simulink model "uavPackageDelivery_3UAV_photo3D_test"  (R2026a)
settings: Solver=VariableStepAuto  StopTime=20  FixedStep=.005  EnableMultiTasking=on
undefined symbols (not defined in the file or in its folder): baseMission, Newton, oaMission, Raphson, uavIC_latLon, UAVSampleTime
libraries: robotcorelib x3, uavalgslib x3, robotalgslib x3, simulink x2
(part 2 of 2)

== system uavPackageDelivery_3UAV_photo3D_test/OnBoard_UAV1/DataProcessing/ProcessSensorData/Compute Ranges/For Each Subsystem ==
  In1 : Inport  Partition=on  PartitionDimension=1  PartitionWidth=1  PartitionOffset=0
  For Each : ForEach  DisableCoverage=on
  Product : Product
  Product1 : Product
  Selector : Selector  InputPortWidth=3  IndexOptions=Index vector (dialog)  Indices=[1]  OutputSizes=1
  Selector1 : Selector  InputPortWidth=3  IndexOptions=Index vector (dialog)  Indices=[2]  OutputSizes=1
  Sqrt : Sqrt  OutputSignalType=real  OutDataTypeStr=single  IntermediateResultsDataTypeStr=single  AlgorithmType=Newton-Raphson
  Sum : Sum  Inputs=|++
  Out1 : Outport  ConcatenationDimension=1
  wires:
  In1/1 -> Selector1/1, Selector/1
  Selector/1 -> Product/2, Product/1
  Selector1/1 -> Product1/2, Product1/1
  Product/1 -> Sum/1
  Product1/1 -> Sum/2
  Sum/1 -> Sqrt/1
  Sqrt/1 -> Out1/1

== system uavPackageDelivery_3UAV_photo3D_test/OnBoard_UAV2/DataProcessing/Process3DSensorData/Compute Ranges/For Each Subsystem1 ==
  In1 : Inport  Partition=on  PartitionDimension=1  PartitionWidth=1  PartitionOffset=0
  For Each Horizontal Slice : ForEach  DisableCoverage=on
  Process each Horizontal Slice : Subsystem  TreatAsAtomicUnit=on
  Reshape : Reshape
  Out1 : Outport  ConcatenationDimension=1
  wires:
  In1/1 -> Process each Horizontal Slice/1(pointCloud)
  Process each Horizontal Slice/1(Out1) -> Reshape/1
  Reshape/1 -> Out1/1

== system uavPackageDelivery_3UAV_photo3D_test/OnBoard_UAV2/DataProcessing/ProcessSensorData/Compute Ranges/For Each Subsystem ==
  In1 : Inport  Partition=on  PartitionDimension=1  PartitionWidth=1  PartitionOffset=0
  For Each : ForEach  DisableCoverage=on
  Product : Product
  Product1 : Product
  Selector : Selector  InputPortWidth=3  IndexOptions=Index vector (dialog)  Indices=[1]  OutputSizes=1
  Selector1 : Selector  InputPortWidth=3  IndexOptions=Index vector (dialog)  Indices=[2]  OutputSizes=1
  Sqrt : Sqrt  OutputSignalType=real  OutDataTypeStr=single  IntermediateResultsDataTypeStr=single  AlgorithmType=Newton-Raphson
  Sum : Sum  Inputs=|++
  Out1 : Outport  ConcatenationDimension=1
  wires:
  In1/1 -> Selector1/1, Selector/1
  Selector/1 -> Product/2, Product/1
  Selector1/1 -> Product1/2, Product1/1
  Product/1 -> Sum/1
  Product1/1 -> Sum/2
  Sum/1 -> Sqrt/1
  Sqrt/1 -> Out1/1

== system uavPackageDelivery_3UAV_photo3D_test/OnBoard_UAV3/DataProcessing/Process3DSensorData/Compute Ranges/For Each Subsystem1 ==
  In1 : Inport  Partition=on  PartitionDimension=1  PartitionWidth=1  PartitionOffset=0
  For Each Horizontal Slice : ForEach  DisableCoverage=on
  Process each Horizontal Slice : Subsystem  TreatAsAtomicUnit=on
  Reshape : Reshape
  Out1 : Outport  ConcatenationDimension=1
  wires:
  In1/1 -> Process each Horizontal Slice/1(pointCloud)
  Process each Horizontal Slice/1(Out1) -> Reshape/1
  Reshape/1 -> Out1/1

== system uavPackageDelivery_3UAV_photo3D_test/OnBoard_UAV3/DataProcessing/ProcessSensorData/Compute Ranges/For Each Subsystem ==
  In1 : Inport  Partition=on  PartitionDimension=1  PartitionWidth=1  PartitionOffset=0
  For Each : ForEach  DisableCoverage=on
  Product : Product
  Product1 : Product
  Selector : Selector  InputPortWidth=3  IndexOptions=Index vector (dialog)  Indices=[1]  OutputSizes=1
  Selector1 : Selector  InputPortWidth=3  IndexOptions=Index vector (dialog)  Indices=[2]  OutputSizes=1
  Sqrt : Sqrt  OutputSignalType=real  OutDataTypeStr=single  IntermediateResultsDataTypeStr=single  AlgorithmType=Newton-Raphson
  Sum : Sum  Inputs=|++
  Out1 : Outport  ConcatenationDimension=1
  wires:
  In1/1 -> Selector1/1, Selector/1
  Selector/1 -> Product/2, Product/1
  Selector1/1 -> Product1/2, Product1/1
  Product/1 -> Sum/1
  Product1/1 -> Sum/2
  Sum/1 -> Sqrt/1
  Sqrt/1 -> Out1/1

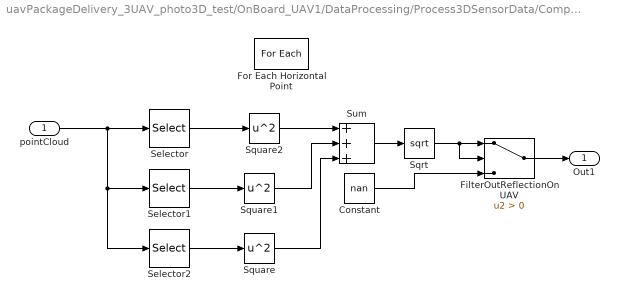
== system uavPackageDelivery_3UAV_photo3D_test/OnBoard_UAV1/DataProcessing/Process3DSensorData/Compute Ranges/For Each Subsystem1/Process each Horizontal Slice ==
  pointCloud : Inport  Partition=on  PartitionDimension=2  PartitionWidth=1  PartitionOffset=0
  Constant : Constant  Value=nan
  FilterOutReflectionOnUAV : Switch  Criteria=u2 > Threshold  SaturateOnIntegerOverflow=off  InputSameDT=off
  For Each Horizontal Point : ForEach  DisableCoverage=on
  Selector : Selector  NumberOfDimensions=3  InputPortWidth=3  IndexOptions=Index vector (dialog),Index vector (dialog),Index vector (dialog)  Indices=1,1,1  OutputSizes=1,1,1
  Selector1 : Selector  NumberOfDimensions=3  InputPortWidth=3  IndexOptions=Index vector (dialog),Index vector (dialog),Index vector (dialog)  Indices=1,1,2  OutputSizes=1,1,1
  Selector2 : Selector  NumberOfDimensions=3  InputPortWidth=3  IndexOptions=Index vector (dialog),Index vector (dialog),Index vector (dialog)  Indices=1,1,3  OutputSizes=1,1,1
  Sqrt : Sqrt  OutputSignalType=real  OutDataTypeStr=single  IntermediateResultsDataTypeStr=single  AlgorithmType=Newton-Raphson
  Square : Math  Operator=square
  Square1 : Math  Operator=square
  Square2 : Math  Operator=square
  Sum : Sum  Inputs=+++
  Out1 : Outport  ConcatenationDimension=1
  wires:
  pointCloud/1 -> Selector2/1, Selector1/1, Selector/1
  Selector/1 -> Square2/1
  Selector1/1 -> Square1/1
  Square2/1 -> Sum/1
  Square1/1 -> Sum/2
  Sum/1 -> Sqrt/1
  Sqrt/1 -> FilterOutReflectionOnUAV/1, FilterOutReflectionOnUAV/2
  Selector2/1 -> Square/1
  Square/1 -> Sum/3
  FilterOutReflectionOnUAV/1 -> Out1/1
  Constant/1 -> FilterOutReflectionOnUAV/3

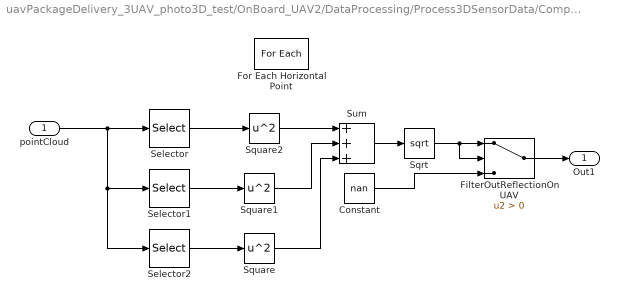
== system uavPackageDelivery_3UAV_photo3D_test/OnBoard_UAV2/DataProcessing/Process3DSensorData/Compute Ranges/For Each Subsystem1/Process each Horizontal Slice ==
  pointCloud : Inport  Partition=on  PartitionDimension=2  PartitionWidth=1  PartitionOffset=0
  Constant : Constant  Value=nan
  FilterOutReflectionOnUAV : Switch  Criteria=u2 > Threshold  SaturateOnIntegerOverflow=off  InputSameDT=off
  For Each Horizontal Point : ForEach  DisableCoverage=on
  Selector : Selector  NumberOfDimensions=3  InputPortWidth=3  IndexOptions=Index vector (dialog),Index vector (dialog),Index vector (dialog)  Indices=1,1,1  OutputSizes=1,1,1
  Selector1 : Selector  NumberOfDimensions=3  InputPortWidth=3  IndexOptions=Index vector (dialog),Index vector (dialog),Index vector (dialog)  Indices=1,1,2  OutputSizes=1,1,1
  Selector2 : Selector  NumberOfDimensions=3  InputPortWidth=3  IndexOptions=Index vector (dialog),Index vector (dialog),Index vector (dialog)  Indices=1,1,3  OutputSizes=1,1,1
  Sqrt : Sqrt  OutputSignalType=real  OutDataTypeStr=single  IntermediateResultsDataTypeStr=single  AlgorithmType=Newton-Raphson
  Square : Math  Operator=square
  Square1 : Math  Operator=square
  Square2 : Math  Operator=square
  Sum : Sum  Inputs=+++
  Out1 : Outport  ConcatenationDimension=1
  wires:
  pointCloud/1 -> Selector2/1, Selector1/1, Selector/1
  Selector/1 -> Square2/1
  Selector1/1 -> Square1/1
  Square2/1 -> Sum/1
  Square1/1 -> Sum/2
  Sum/1 -> Sqrt/1
  Sqrt/1 -> FilterOutReflectionOnUAV/1, FilterOutReflectionOnUAV/2
  Selector2/1 -> Square/1
  Square/1 -> Sum/3
  FilterOutReflectionOnUAV/1 -> Out1/1
  Constant/1 -> FilterOutReflectionOnUAV/3

== system uavPackageDelivery_3UAV_photo3D_test/OnBoard_UAV3/DataProcessing/Process3DSensorData/Compute Ranges/For Each Subsystem1/Process each Horizontal Slice ==
  pointCloud : Inport  Partition=on  PartitionDimension=2  PartitionWidth=1  PartitionOffset=0
  Constant : Constant  Value=nan
  FilterOutReflectionOnUAV : Switch  Criteria=u2 > Threshold  SaturateOnIntegerOverflow=off  InputSameDT=off
  For Each Horizontal Point : ForEach  DisableCoverage=on
  Selector : Selector  NumberOfDimensions=3  InputPortWidth=3  IndexOptions=Index vector (dialog),Index vector (dialog),Index vector (dialog)  Indices=1,1,1  OutputSizes=1,1,1
  Selector1 : Selector  NumberOfDimensions=3  InputPortWidth=3  IndexOptions=Index vector (dialog),Index vector (dialog),Index vector (dialog)  Indices=1,1,2  OutputSizes=1,1,1
  Selector2 : Selector  NumberOfDimensions=3  InputPortWidth=3  IndexOptions=Index vector (dialog),Index vector (dialog),Index vector (dialog)  Indices=1,1,3  OutputSizes=1,1,1
  Sqrt : Sqrt  OutputSignalType=real  OutDataTypeStr=single  IntermediateResultsDataTypeStr=single  AlgorithmType=Newton-Raphson
  Square : Math  Operator=square
  Square1 : Math  Operator=square
  Square2 : Math  Operator=square
  Sum : Sum  Inputs=+++
  Out1 : Outport  ConcatenationDimension=1
  wires:
  pointCloud/1 -> Selector2/1, Selector1/1, Selector/1
  Selector/1 -> Square2/1
  Selector1/1 -> Square1/1
  Square2/1 -> Sum/1
  Square1/1 -> Sum/2
  Sum/1 -> Sqrt/1
  Sqrt/1 -> FilterOutReflectionOnUAV/1, FilterOutReflectionOnUAV/2
  Selector2/1 -> Square/1
  Square/1 -> Sum/3
  FilterOutReflectionOnUAV/1 -> Out1/1
  Constant/1 -> FilterOutReflectionOnUAV/3

== matlab function uavPackageDelivery_3UAV_photo3D_test/GroundControl_UAV2/Get Flight Mission/QGC/Create Mission for Path Manager ==
  data: baseMission input Bus: uavPathManagerBus size=42; isNew input size=1; LTPMission input size=[42 3]; mission output Bus: uavPathManagerBus size=42; qgcMission input Bus: uavPathManagerBus size=42
function mission = generateWaypointStream(baseMission, isNew, LTPMission, qgcMission)

persistent UAVMission

if isempty(UAVMission)
    UAVMission = baseMission;
end

%% If we got a new mission
if (isNew == true)
   for ii=1:42
       if LTPMission(ii,2) < 7275326
           UAVMission(ii).position = LTPMission(ii,:)';
           y = isnan(qgcMission(ii).params);
           UAVMission(ii).params = qgcMission(ii).params;
           if sum(y)>0
               UAVMission(ii).params(y) = single(0);
           end
           UAVMission(ii).mode = mavlinkToPlannerType(qgcMission(ii).mode);
       end
   end
end

mission = UAVMission;

end

function plannerType =  mavlinkToPlannerType (mavlinkType)
% see enum name="MAV_CMD" in common.xml for values.
    switch mavlinkType
        case 16 %MAV_CMD_NAV_WAYPOINT
            plannerType = uint8(2);
        case 18 %MAV_CMD_NAV_LOITER_TURNS
            plannerType = uint8(3);
        case 21 %MAV_CMD_NAV_LAND
            plannerType = uint8(4);
        case 22 %MAV_CMD_NAV_TAKEOFF
            plannerType = uint8(1);
        otherwise %this will likely error out to signal something unexpected
            plannerType = uint8(0);
    end
end

== matlab function uavPackageDelivery_3UAV_photo3D_test/OnBoard_UAV2/DataProcessing/Process3DSensorData/ObstacleAvoidance/ReshapePointCloud ==
  data: u input; y output
function y = fcn(u)
y = [reshape(u(:,:,1),[],1), reshape(u(:,:,2),[],1), reshape(u(:,:,3),[],1)];

== matlab function uavPackageDelivery_3UAV_photo3D_test/OnBoard_UAV2/DataProcessing/Process3DSensorData/Visualize Front-Facing Camera ==
  data: imageFrame input
function plotImageFrame(imageFrame)

coder.extrinsic('ishandle','image');

persistent fig;

if isempty(fig)
    fig = figure();
    ax = newplot(fig);
    title(ax, 'Front-facing camera');
end

if ~isempty(fig) && ishandle(fig)
    ax = newplot(fig);
    image(ax, imageFrame);
    axis(ax, 'off');
end

== matlab function uavPackageDelivery_3UAV_photo3D_test/OnBoard_UAV2/DataProcessing/Process3DSensorData/Visualize Point cloud ==
  data: xyzPoints input
function VisualizePointCloud(xyzPoints)
%VisualizePointCloud Display point cloud

coder.extrinsic('isOpen', 'pcplayer')

persistent player;

if isempty(player)
    % Configure axes limits
    xlimits = [-90 90];
    ylimits = [-90 90];
    zlimits = [ -50 50];
    
    % Create a streaming Lidar viewer
    player = pcplayer(xlimits, ylimits, zlimits);
end

if ~isempty(player) && isOpen(player)
    view(player, xyzPoints);
end

== matlab function uavPackageDelivery_3UAV_photo3D_test/OnBoard_UAV2/DataProcessing/ProcessSensorData/Target Direction calculator ==
  data: u input; Dir output; pos input
function Dir = TargetDir(u, pos)

Dir = atan2(u(2)-pos.y, u(1)-pos.x);

end

== matlab function uavPackageDelivery_3UAV_photo3D_test/OnBoard_UAV2/DataProcessing/ProcessSensorData/Visualize Front-Facing Camera ==
  data: imageFrame input
function plotImageFrame(imageFrame)

coder.extrinsic('ishandle','image');

persistent fig;

if isempty(fig)
    fig = figure();
    ax = newplot(fig);
    title(ax, 'Front-facing camera');
end

if ~isempty(fig) && ishandle(fig)
    ax = newplot(fig);
    image(ax, imageFrame);
    axis(ax, 'off');
end

== matlab function uavPackageDelivery_3UAV_photo3D_test/OnBoard_UAV2/DataProcessing/ProcessSensorData/Visualize Point cloud ==
  data: xyzPoints input
function VisualizePointCloud(xyzPoints)
%VisualizePointCloud Display point cloud

coder.extrinsic('isOpen', 'pcplayer')

persistent player;

if isempty(player)
    % Configure axes limits
    xlimits = [-90 90];
    ylimits = [-90 90];
    zlimits = [ -50 50];
    
    % Create a streaming Lidar viewer
    player = pcplayer(xlimits, ylimits, zlimits);
end

if ~isempty(player) && isOpen(player)
    view(player, xyzPoints);
end

== matlab function uavPackageDelivery_3UAV_photo3D_test/OnBoard_UAV3/DataProcessing/Process3DSensorData/ObstacleAvoidance/ReshapePointCloud ==
  data: u input; y output
function y = fcn(u)
y = [reshape(u(:,:,1),[],1), reshape(u(:,:,2),[],1), reshape(u(:,:,3),[],1)];

== matlab function uavPackageDelivery_3UAV_photo3D_test/OnBoard_UAV3/DataProcessing/Process3DSensorData/Visualize Front-Facing Camera ==
  data: imageFrame input
function plotImageFrame(imageFrame)

coder.extrinsic('ishandle','image');

persistent fig;

if isempty(fig)
    fig = figure();
    ax = newplot(fig);
    title(ax, 'Front-facing camera');
end

if ~isempty(fig) && ishandle(fig)
    ax = newplot(fig);
    image(ax, imageFrame);
    axis(ax, 'off');
end

== matlab function uavPackageDelivery_3UAV_photo3D_test/OnBoard_UAV3/DataProcessing/Process3DSensorData/Visualize Point cloud ==
  data: xyzPoints input
function VisualizePointCloud(xyzPoints)
%VisualizePointCloud Display point cloud

coder.extrinsic('isOpen', 'pcplayer')

persistent player;

if isempty(player)
    % Configure axes limits
    xlimits = [-90 90];
    ylimits = [-90 90];
    zlimits = [ -50 50];
    
    % Create a streaming Lidar viewer
    player = pcplayer(xlimits, ylimits, zlimits);
end

if ~isempty(player) && isOpen(player)
    view(player, xyzPoints);
end

== matlab function uavPackageDelivery_3UAV_photo3D_test/OnBoard_UAV3/DataProcessing/ProcessSensorData/Target Direction calculator ==
  data: u input; Dir output; pos input
function Dir = TargetDir(u, pos)

Dir = atan2(u(2)-pos.y, u(1)-pos.x);

end

== matlab function uavPackageDelivery_3UAV_photo3D_test/OnBoard_UAV3/DataProcessing/ProcessSensorData/Visualize Front-Facing Camera ==
  data: imageFrame input
function plotImageFrame(imageFrame)

coder.extrinsic('ishandle','image');

persistent fig;

if isempty(fig)
    fig = figure();
    ax = newplot(fig);
    title(ax, 'Front-facing camera');
end

if ~isempty(fig) && ishandle(fig)
    ax = newplot(fig);
    image(ax, imageFrame);
    axis(ax, 'off');
end

== matlab function uavPackageDelivery_3UAV_photo3D_test/OnBoard_UAV3/DataProcessing/ProcessSensorData/Visualize Point cloud ==
  data: xyzPoints input
function VisualizePointCloud(xyzPoints)
%VisualizePointCloud Display point cloud

coder.extrinsic('isOpen', 'pcplayer')

persistent player;

if isempty(player)
    % Configure axes limits
    xlimits = [-90 90];
    ylimits = [-90 90];
    zlimits = [ -50 50];
    
    % Create a streaming Lidar viewer
    player = pcplayer(xlimits, ylimits, zlimits);
end

if ~isempty(player) && isOpen(player)
    view(player, xyzPoints);
end

== matlab function uavPackageDelivery_3UAV_photo3D_test/OnBoard_UAV1/DataProcessing/ProcessSensorData/Visualize Front-Facing Camera ==
  data: imageFrame input
function plotImageFrame(imageFrame)

coder.extrinsic('ishandle','image');

persistent fig;

if isempty(fig)
    fig = figure();
    ax = newplot(fig);
    title(ax, 'Front-facing camera');
end

if ~isempty(fig) && ishandle(fig)
    ax = newplot(fig);
    image(ax, imageFrame);
    axis(ax, 'off');
end

== matlab function uavPackageDelivery_3UAV_photo3D_test/OnBoard_UAV1/DataProcessing/Process3DSensorData/ObstacleAvoidance/ReshapePointCloud ==
  data: u input; y output
function y = fcn(u)
y = [reshape(u(:,:,1),[],1), reshape(u(:,:,2),[],1), reshape(u(:,:,3),[],1)];

== matlab function uavPackageDelivery_3UAV_photo3D_test/OnBoard_UAV1/DataProcessing/Process3DSensorData/Visualize Front-Facing Camera ==
  data: imageFrame input
function plotImageFrame(imageFrame)

coder.extrinsic('ishandle','image');

persistent fig;

if isempty(fig)
    fig = figure();
    ax = newplot(fig);
    title(ax, 'Front-facing camera');
end

if ~isempty(fig) && ishandle(fig)
    ax = newplot(fig);
    image(ax, imageFrame);
    axis(ax, 'off');
end

== matlab function uavPackageDelivery_3UAV_photo3D_test/OnBoard_UAV1/DataProcessing/Process3DSensorData/Visualize Point cloud ==
  data: xyzPoints input
function VisualizePointCloud(xyzPoints)
%VisualizePointCloud Display point cloud

coder.extrinsic('isOpen', 'pcplayer')

persistent player;

if isempty(player)
    % Configure axes limits
    xlimits = [-90 90];
    ylimits = [-90 90];
    zlimits = [ -50 50];
    
    % Create a streaming Lidar viewer
    player = pcplayer(xlimits, ylimits, zlimits);
end

if ~isempty(player) && isOpen(player)
    view(player, xyzPoints);
end

== matlab function uavPackageDelivery_3UAV_photo3D_test/GroundControl_UAV1/Get Flight Mission/QGC/Mission to Xe/MATLAB Function ==
  data: mission input Bus: uavPathManagerBus size=42; waypoints output single size=[42 3]
function waypoints  = buildUAVMission(mission)
%
waypoints = single(zeros(42,3));

for i=1:length(mission)
    waypoints(i,1:3) = mission(i).position;
end

end

== matlab function uavPackageDelivery_3UAV_photo3D_test/GroundControl_UAV1/Get Flight Mission/QGC/Create Mission for Path Manager ==
  data: baseMission input Bus: uavPathManagerBus size=42; isNew input size=1; LTPMission input size=[42 3]; mission output Bus: uavPathManagerBus size=42; qgcMission input Bus: uavPathManagerBus size=42
function mission = generateWaypointStream(baseMission, isNew, LTPMission, qgcMission)

persistent UAVMission

if isempty(UAVMission)
    UAVMission = baseMission;
end

%% If we got a new mission
if (isNew == true)
   for ii=1:42
       if LTPMission(ii,2) < 7275326
           UAVMission(ii).position = LTPMission(ii,:)';
           y = isnan(qgcMission(ii).params);
           UAVMission(ii).params = qgcMission(ii).params;
           if sum(y)>0
               UAVMission(ii).params(y) = single(0);
           end
           UAVMission(ii).mode = mavlinkToPlannerType(qgcMission(ii).mode);
       end
   end
end

mission = UAVMission;

end

function plannerType =  mavlinkToPlannerType (mavlinkType)
% see enum name="MAV_CMD" in common.xml for values.
    switch mavlinkType
        case 16 %MAV_CMD_NAV_WAYPOINT
            plannerType = uint8(2);
        case 18 %MAV_CMD_NAV_LOITER_TURNS
            plannerType = uint8(3);
        case 21 %MAV_CMD_NAV_LAND
            plannerType = uint8(4);
        case 22 %MAV_CMD_NAV_TAKEOFF
            plannerType = uint8(1);
        otherwise %this will likely error out to signal something unexpected
            plannerType = uint8(0);
    end
end

== matlab function uavPackageDelivery_3UAV_photo3D_test/OnBoard_UAV1/DataProcessing/ProcessSensorData/Target Direction calculator ==
  data: u input; Dir output; pos input
function Dir = TargetDir(u, pos)

Dir = atan2(u(2)-pos.y, u(1)-pos.x);

end

== matlab function uavPackageDelivery_3UAV_photo3D_test/GroundControl_UAV2/Get Flight Mission/QGC/Mission to Xe/MATLAB Function ==
  data: mission input Bus: uavPathManagerBus size=42; waypoints output single size=[42 3]
function waypoints  = buildUAVMission(mission)
%
waypoints = single(zeros(42,3));

for i=1:length(mission)
    waypoints(i,1:3) = mission(i).position;
end

end

== matlab function uavPackageDelivery_3UAV_photo3D_test/OnBoard_UAV1/DataProcessing/ProcessSensorData/Visualize Point cloud ==
  data: xyzPoints input
function VisualizePointCloud(xyzPoints)
%VisualizePointCloud Display point cloud

coder.extrinsic('isOpen', 'pcplayer')

persistent player;

if isempty(player)
    % Configure axes limits
    xlimits = [-90 90];
    ylimits = [-90 90];
    zlimits = [ -50 50];
    
    % Create a streaming Lidar viewer
    player = pcplayer(xlimits, ylimits, zlimits);
end

if ~isempty(player) && isOpen(player)
    view(player, xyzPoints);
end

== matlab function uavPackageDelivery_3UAV_photo3D_test/GroundControl_UAV3/Get Flight Mission/QGC/Create Mission for Path Manager ==
  data: baseMission input Bus: uavPathManagerBus size=42; isNew input size=1; LTPMission input size=[42 3]; mission output Bus: uavPathManagerBus size=42; qgcMission input Bus: uavPathManagerBus size=42
function mission = generateWaypointStream(baseMission, isNew, LTPMission, qgcMission)

persistent UAVMission

if isempty(UAVMission)
    UAVMission = baseMission;
end

%% If we got a new mission
if (isNew == true)
   for ii=1:42
       if LTPMission(ii,2) < 7275326
           UAVMission(ii).position = LTPMission(ii,:)';
           y = isnan(qgcMission(ii).params);
           UAVMission(ii).params = qgcMission(ii).params;
           if sum(y)>0
               UAVMission(ii).params(y) = single(0);
           end
           UAVMission(ii).mode = mavlinkToPlannerType(qgcMission(ii).mode);
       end
   end
end

mission = UAVMission;

end

function plannerType =  mavlinkToPlannerType (mavlinkType)
% see enum name="MAV_CMD" in common.xml for values.
    switch mavlinkType
        case 16 %MAV_CMD_NAV_WAYPOINT
            plannerType = uint8(2);
        case 18 %MAV_CMD_NAV_LOITER_TURNS
            plannerType = uint8(3);
        case 21 %MAV_CMD_NAV_LAND
            plannerType = uint8(4);
        case 22 %MAV_CMD_NAV_TAKEOFF
            plannerType = uint8(1);
        otherwise %this will likely error out to signal something unexpected
            plannerType = uint8(0);
    end
end

== matlab function uavPackageDelivery_3UAV_photo3D_test/GroundControl_UAV3/Get Flight Mission/QGC/Mission to Xe/MATLAB Function ==
  data: mission input Bus: uavPathManagerBus size=42; waypoints output single size=[42 3]
function waypoints  = buildUAVMission(mission)
%
waypoints = single(zeros(42,3));

for i=1:length(mission)
    waypoints(i,1:3) = mission(i).position;
end

end
